simulink model "BDA_DynamicModel"  (R2021b)
settings: Solver=ode23t  StartTime=0.0  StopTime=10  FixedStep=0.000001  MaxStep=1e-5  MinStep=1e-7  RelTol=1e-3
undefined symbols (not defined in the file or in its folder): X, Y, Z
libraries: sm_lib x47, nesl_utility x7
(part 3 of 3)

== matlab function BDA_DynamicModel/H ==
  data: q2 input; H output; q3 input; q4 input; q5 input; q6 input
function H = H(q2,q3,q4,q5,q6)
%#codegen

%    This function was generated by the Symbolic Math Toolbox version 9.0.
%    01-Nov-2021 22:23:37

t2 = conj(q2);
t3 = conj(q3);
t4 = conj(q4);
t5 = conj(q5);
t6 = conj(q6);
t7 = cos(q2);
t8 = cos(q4);
t9 = cos(q5);
t10 = cos(q6);
t11 = sin(q2);
t12 = sin(q4);
t13 = sin(q5);
t14 = sin(q6);
t33 = 9.007199254740992e+15;
t15 = cos(t2);
t16 = cos(t4);
t17 = cos(t5);
t18 = cos(t6);
t19 = sin(t2);
t20 = sin(t4);
t21 = sin(t5);
t22 = sin(t6);
t25 = t7.*1.051339e-1;
t26 = t11.*1.051339e-1;
t27 = t9.*5.110348748545983e-1;
t29 = t13.*5.110348748545983e-1;
t32 = t11.*3.235525e-2;
t37 = t7.*3.235525e-2;
t40 = t9.*t12.*8.595599785252598e-1;
t41 = t12.*t13.*8.595599785252598e-1;
t55 = t9.*5.7e-7;
t56 = t10.*9.3e-7;
t57 = t14.*1.02e-6;
t63 = t13.*2.4e-7;
t65 = t9.*t14.*9.3e-7;
t66 = t14.*9.0e-8;
t67 = t13.*5.110348748545983e-9;
t68 = t10.*t13.*4.36041e-5;
t69 = t13.*t14.*4.36041e-5;
t70 = t9.*4.0e-8;
t71 = t13.*4.0e-8;
t72 = t10.*9.0e-8;
t73 = t9.*t10.*1.02e-6;
t75 = t8.*8.595599785252598e-9;
t79 = t9.*t12.*8.595599785252598e-9;
t82 = (q3.*t33)./9.007199254740992e+15;
t83 = (t3.*t33)./9.007199254740992e+15;
t88 = q3.*t33.*1.110223024625157e-16i;
t89 = t3.*t33.*1.110223024625157e-16i;
t114 = t10.*1.33637554986e-4;
t115 = t13.*1.33637554986e-4;
t117 = t13.*7.26350557185e-5;
t118 = t14.*7.26350557185e-5;
t119 = t13.*6.1855407534e-5;
t123 = t9.*1.35652563578e-4;
t127 = t9.*2.912898786671211e-7;
t131 = t8.*5.329271866856611e-7;
t134 = t9.*t10.*7.26350557185e-5;
t135 = t8.*2.784974330421842e-6;
t136 = t13.*5.212555723516903e-7;
t138 = t8.*6.730354631852784e-6;
t139 = t8.*3.748033925961328e-5;
t140 = t9.*t14.*1.33637554986e-4;
t150 = t13.*1.226483699651036e-7;
t151 = t9.*2.044139499418393e-8;
t152 = t13.*2.044139499418393e-8;
t156 = t12.*t13.*4.899491877593981e-7;
t158 = t8.*t10.*7.993907800284916e-7;
t161 = t9.*t12.*8.76751178095765e-7;
t162 = t8.*t14.*8.76751178095765e-7;
t163 = t9.*t12.*2.062943948460623e-7;
t169 = t9.*t12.*3.438239914101039e-8;
t171 = t12.*t13.*3.438239914101039e-8;
t172 = t8.*t10.*7.736039806727338e-8;
t173 = t8.*t14.*7.736039806727338e-8;
t211 = t13.*3.161027044821787e-5;
t213 = t13.*3.711904660916042e-5;
t214 = t9.*6.932319085178867e-5;
t215 = t8.*9.395517395143932e-4;
t216 = t12.*9.395517395143932e-4;
t217 = t9.*3.601891949238275e-7;
t218 = t13.*3.601891949238275e-7;
t219 = t8.*5.316843277159623e-5;
t220 = t12.*1.451749445763287e-4;
t222 = t8.*1.166015146360021e-4;
t224 = t13.*6.829345118814501e-5;
t227 = t12.*5.427853659906482e-4;
t228 = t8.*t10.*1.148694938939344e-4;
t229 = t9.*t12.*6.243418693357491e-5;
t230 = t8.*t14.*6.243418693357491e-5;
t231 = t9.*t12.*1.148694938939344e-4;
t232 = t9.*t12.*5.316843277159623e-5;
t233 = t12.*t13.*1.166015146360021e-4;
t234 = t8.*t9.*5.427853659906482e-4;
t235 = t8.*t13.*5.427853659906482e-4;
t236 = t9.*t12.*6.058377458913066e-7;
t237 = t12.*t13.*6.058377458913066e-7;
t238 = t8.*1.607033050476913e-7;
t239 = t8.*t9.*3.626595104792852e-4;
t240 = t10.*t12.*3.626595104792852e-4;
t241 = t12.*t14.*3.626595104792852e-4;
t243 = t8.*t10.*t13.*3.626595104792852e-4;
t244 = t8.*t13.*t14.*3.626595104792852e-4;
t23 = t18.*t21.*(3.0./5.0e+2);
t24 = t21.*t22.*(3.0./5.0e+2);
t28 = -t26;
t30 = t15.*1.051339e-1;
t31 = t19.*1.051339e-1;
t34 = t17.*5.110348748545983e-1;
t36 = t21.*5.110348748545983e-1;
t38 = t15.*3.235525e-2;
t39 = t19.*3.235525e-2;
t42 = t21.*9.99471e-3;
t43 = t22.*9.99471e-3;
t44 = t18.*1.838876e-2;
t45 = t21.*1.838876e-2;
t46 = t17.*1.247162e-2;
t47 = t21.*5.68686e-3;
t48 = -t41;
t50 = t16.*5.157359871151559e-3;
t51 = t16.*t18.*8.595599785252598e-1;
t52 = t17.*t20.*8.595599785252598e-1;
t53 = t16.*t22.*8.595599785252598e-1;
t54 = t20.*t21.*8.595599785252598e-1;
t58 = t17.*t18.*9.99471e-3;
t59 = t17.*t22.*1.838876e-2;
t62 = -t57;
t74 = -t66;
t76 = -t75;
t77 = t9.*t72;
t78 = t9.*t66;
t84 = cos(t82);
t85 = sin(t82);
t86 = cos(t83);
t87 = sin(t83);
t90 = exp(t88);
t91 = -t88;
t92 = -t89;
t96 = exp(t89);
t105 = t17.*6.373432765934105e-3;
t106 = t21.*5.107645374058002e-3;
t107 = t21.*2.906183788415621e-3;
t108 = t16.*3.251444605336828e-2;
t109 = t20.*3.251444605336828e-2;
t110 = t16.*1.07201054193752e-2;
t111 = t21.*9.397297665331243e-3;
t112 = t21.*3.311505989057797e-5;
t116 = t16.*4.888197259476159e-3;
t120 = t20.*5.023973353684009e-3;
t121 = t20.*4.990257941055339e-2;
t122 = t17.*3.311505989057797e-5;
t125 = t25+t32;
t126 = -t119;
t130 = t16.*t18.*1.580624215070616e-2;
t132 = t20.*t21.*1.07201054193752e-2;
t133 = t17.*t20.*1.580624215070616e-2;
t141 = t17.*t20.*8.5910527129662e-3;
t142 = t16.*t22.*8.5910527129662e-3;
t143 = t16.*t21.*4.990257941055339e-2;
t145 = -t131;
t148 = t16.*5.561353061058431e-6;
t149 = t17.*t20.*4.888197259476159e-3;
t153 = t16.*t17.*4.990257941055339e-2;
t154 = -t140;
t157 = t29+t40;
t159 = t17.*t20.*5.569948660843684e-5;
t160 = t20.*t21.*5.569948660843684e-5;
t164 = -t156;
t167 = -t162;
t174 = t16.*t18.*t21.*(-4.990257941055339e-2);
t175 = -t171;
t177 = -t173;
t184 = t55+t71;
t187 = t63+t70;
t223 = -t214;
t225 = -t217;
t226 = -t218;
t242 = -t236;
t245 = -t243;
t246 = t69+t117;
t247 = t68+t115;
t282 = t135+1.589318460797801e-6;
t283 = t138+1.655752994528898e-6;
t300 = t136+t161;
t338 = t114+t118+4.36041e-5;
t380 = t215-8.631097478604537e-5;
t381 = t216+9.554306323645785e-8;
t384 = t220+t238;
t35 = -t31;
t49 = -t47;
t60 = -t53;
t61 = -t54;
t64 = -t59;
t80 = t24+t42;
t81 = t23+t45;
t93 = 1.0./t90;
t94 = t8.*t84;
t95 = t12.*t84;
t97 = exp(t92);
t98 = t16.*t86;
t99 = t20.*t86;
t100 = t90-1.0;
t113 = -t105;
t124 = -t112;
t129 = -t122;
t137 = t28+t37;
t144 = t18.*t121;
t146 = t22.*t121;
t147 = t30+t39;
t165 = t27+t48;
t166 = -t159;
t168 = t18.*t143;
t170 = t22.*t143;
t176 = t36+t52;
t180 = t43+t44+3.0./5.0e+2;
t188 = t56+t74;
t189 = t62+t72;
t190 = t65+t77;
t191 = t73+t78;
t192 = t84.*1.273194e-2;
t193 = t86.*1.273194e-2;
t194 = t86.*1.025512e-2;
t196 = t86.*9.224950000000001e-3;
t248 = t10.*t157.*4.36041e-5;
t249 = t14.*t157.*4.36041e-5;
t258 = t84.*3.42298471896e-5;
t260 = t84.*3.07913148585e-5;
t261 = t90.*3.694216783411725e-1;
t262 = t90.*1.305783216588275e-1;
t264 = t84.*3.679077402936e-4;
t265 = t96.*1.305783216588275e-1;
t266 = t96.*3.694216783411725e-1;
t280 = t108-2.986906857247653e-3;
t281 = t109+3.306395640309251e-6;
t284 = t123+t126;
t285 = t120+t148;
t286 = t8.*t33.*t85.*5.673626844500105e-17;
t287 = t12.*t33.*t85.*5.673626844500105e-17;
t288 = t9.*t33.*t85.*9.543032792050485e-17;
t289 = t13.*t33.*t85.*9.543032792050485e-17;
t294 = t134+t154;
t296 = t16.*t33.*t87.*5.673626844500105e-17;
t297 = t20.*t33.*t87.*5.673626844500105e-17;
t298 = t17.*t33.*t87.*9.543032792050485e-17;
t299 = t21.*t33.*t87.*9.543032792050485e-17;
t303 = t16.*t33.*t87.*3.404176106700063e-19;
t304 = t8.*t33.*t85.*5.673626844500105e-25;
t305 = t13.*t33.*t85.*9.543032792050485e-25;
t306 = t84.*t86.*2.2e-7;
t307 = t90.*3.215186923359161e-3;
t309 = t90.*1.345257168956303e-2;
t310 = t96.*3.215186923359161e-3;
t311 = t96.*1.345257168956303e-2;
t319 = t67+t79+t145;
t322 = t33.*t85.*4.87211480085e-18;
t323 = t33.*t87.*4.87211480085e-18;
t324 = t33.*t87.*6.374153504905841e-18;
t325 = t12.*t33.*t85.*5.582848814988104e-22;
t327 = t33.*t87.*5.577730892363251e-19;
t328 = t8.*t33.*t85.*2.479366200131245e-18;
t329 = t21.*t33.*t87.*9.537984527703491e-19;
t330 = t8.*t33.*t85.*7.351481000981246e-18;
t331 = t8.*t33.*t85.*4.442449819243582e-22;
t332 = t12.*t33.*t85.*9.810473427588925e-18;
t333 = t12.*t33.*t85.*4.938358626738924e-18;
t334 = t8.*t33.*t85.*3.517648643590065e-23;
t335 = t33.*t85.*3.091942624624357e-22;
t336 = t16.*t33.*t87.*2.479366200131245e-18;
t337 = t8.*t33.*t85.*1.838255097618034e-22;
t339 = t16.*t33.*t87.*3.226512155691387e-19;
t342 = t21.*t33.*t87.*5.426989146380022e-19;
t343 = t33.*t85.*2.967883198327701e-22;
t344 = t20.*t33.*t87.*3.31613276532711e-19;
t345 = t17.*t33.*t87.*1.190170786299927e-18;
t346 = t21.*t33.*t87.*1.754845396851463e-18;
t348 = t16.*t33.*t87.*7.075931802640439e-19;
t349 = t20.*t33.*t87.*4.938358626738924e-18;
t350 = t33.*t87.*6.174342216456664e-22;
t352 = t16.*t33.*t87.*8.66274921222547e-18;
t354 = t16.*t33.*t87.*3.790634411375469e-18;
t355 = t20.*t33.*t87.*8.66274921222547e-18;
t357 = t20.*t33.*t87.*3.790634411375469e-18;
t358 = t8.*t33.*t85.*2.47393392290267e-21;
t359 = t16.*t33.*t87.*7.351481000981246e-18;
t360 = t20.*t33.*t87.*9.810473427588925e-18;
t362 = t9.*t33.*t85.*5.439528691468777e-23;
t363 = t17.*t33.*t87.*6.183885249248715e-21;
t364 = t21.*t33.*t87.*6.183885249248715e-21;
t365 = t13.*t33.*t85.*9.733893447891495e-23;
t369 = t13.*t33.*t85.*2.290327870092116e-23;
t370 = t16.*t33.*t87.*3.670836568391568e-22;
t372 = t9.*t33.*t85.*3.817213116820194e-24;
t373 = t13.*t33.*t85.*3.817213116820194e-24;
t374 = t90.*1.073174736839591e-5;
t375 = t90.*4.490239736257417e-5;
t378 = t90.*3.887314306731568e-4;
t382 = t33.*t85.*2.127584079327986e-20;
t386 = t33.*t85.*1.611765660673211e-20;
t387 = t13.*t33.*t85.*6.931587185740596e-21;
t388 = t8.*t33.*t85.*7.696420262413979e-21;
t389 = t8.*t33.*t85.*3.509445006623964e-21;
t390 = t9.*t33.*t85.*1.294536862550567e-20;
t391 = t12.*t33.*t85.*5.371403294717661e-20;
t392 = t8.*t33.*t85.*9.394124637620594e-23;
t395 = t13.*t33.*t85.*1.275307569480848e-20;
t397 = t12.*t33.*t85.*9.582443148530891e-21;
t398 = t13.*t33.*t85.*5.902881824626087e-21;
t401 = t9.*t33.*t85.*6.726150146755334e-23;
t402 = t13.*t33.*t85.*6.726150146755334e-23;
t404 = t33.*t85.*1.78416509397307e-23;
t405 = t8.*t33.*t85.*2.503226128461205e-19;
t406 = t12.*t33.*t85.*2.503226128461205e-19;
t407 = t8.*t33.*t85.*1.095358398302466e-19;
t409 = t12.*t33.*t85.*1.06707538424542e-19;
t410 = t12.*t33.*t85.*1.095358398302466e-19;
t415 = t8.*t33.*t85.*1.060741086483328e-23;
t419 = t33.*t85.*t125.*5.673626844500105e-17;
t424 = t85.*t87.*7.913131956031502e-8;
t434 = t13.*t33.*t85.*4.011313864537747e-22;
t435 = t9.*t33.*t85.*3.825067422357704e-25;
t436 = t8.*t33.*t85.*1.511210377393976e-22;
t438 = t33.*t85.*t125.*1.893760189037778e-19;
t439 = t21.*t33.*t87.*4.011313864537747e-22;
t440 = t17.*t33.*t87.*3.825067422357704e-25;
t441 = t16.*t33.*t87.*1.511210377393976e-22;
t471 = t33.*t85.*3.909932369564116e-22;
t472 = t13.*t33.*t85.*1.793163166137816e-24;
t473 = t33.*t87.*3.909932369564116e-22;
t474 = t21.*t33.*t87.*1.793163166137816e-24;
t481 = t33.*t85.*9.467866758889686e-23;
t482 = t33.*t87.*5.699051429514929e-23;
t498 = t33.*t87.*t282.*9.543032792050485e-17;
t505 = t127+t152+t164+t169;
t523 = t76+t150+t151+t163+t175;
t557 = t219+t225+t234+t237;
t558 = t222+t226+t235+t242;
t583 = t211+t223+t227+t232+t233;
t101 = t100.^2;
t102 = t97-1.0;
t104 = t99.*(3.0./5.0e+2);
t128 = t95./1.0e+8;
t155 = t35+t38;
t178 = t34+t61;
t179 = t46+t49;
t183 = t58+t64;
t185 = t18.*t176.*(3.0./5.0e+2);
t186 = t22.*t176.*(3.0./5.0e+2);
t195 = t95.*2.228474e-2;
t197 = t94.*6.562549e-2;
t198 = t94.*9.840000000000001e-6;
t199 = t98.*4.539638e-2;
t200 = t99.*4.539638e-2;
t201 = t99.*1.247162e-2;
t202 = t99.*2.228474e-2;
t203 = t98.*5.84482e-3;
t204 = t98.*6.562549e-2;
t205 = t99.*5.68686e-3;
t207 = t95.*3.24e-6;
t208 = t95.*7.83e-6;
t209 = t95.*4.36041e-5;
t210 = t95.*6.2e-7;
t212 = t99.*6.47e-6;
t251 = t10.*t165.*1.02e-6;
t252 = t14.*t165.*9.3e-7;
t255 = t72.*t165;
t256 = t66.*t165;
t263 = t93.*3.694216783411725e-1;
t267 = t93.*1.305783216588275e-1;
t268 = t97.*1.305783216588275e-1;
t269 = t97.*3.694216783411725e-1;
t270 = t94.*1.3117937708872e-3;
t271 = t95.*1.3117937708872e-3;
t272 = t95.*1.35652563578e-4;
t273 = t94.*1.688944904408e-4;
t274 = t95.*6.1855407534e-5;
t275 = t94.*7.13801892181e-4;
t276 = t95.*1.655752994528898e-6;
t277 = t95.*1.869599668e-7;
t290 = t14.*t165.*1.33637554986e-4;
t291 = t10.*t165.*7.26350557185e-5;
t292 = -t287;
t293 = -t288;
t301 = -t297;
t302 = -t298;
t308 = t93.*3.215186923359161e-3;
t312 = t93.*1.345257168956303e-2;
t313 = t97.*3.215186923359161e-3;
t314 = t97.*1.345257168956303e-2;
t315 = t95.*4.427198467956924e-6;
t316 = t95.*2.663570267859459e-6;
t317 = t99.*4.427198467956924e-6;
t318 = t99.*2.663570267859459e-6;
t320 = t94.*8.487305697640184e-9;
t321 = t98.*8.487305697640184e-9;
t326 = -t325;
t340 = -t332;
t341 = -t333;
t347 = -t335;
t351 = -t343;
t353 = -t344;
t356 = -t345;
t361 = -t349;
t366 = -t355;
t367 = -t357;
t368 = -t360;
t371 = -t370;
t376 = t93.*1.073174736839591e-5;
t377 = t93.*4.490239736257417e-5;
t379 = t93.*3.887314306731568e-4;
t383 = t95+t286;
t396 = t99+t296;
t399 = -t390;
t400 = -t391;
t403 = -t392;
t411 = -t397;
t412 = -t406;
t413 = -t409;
t414 = -t410;
t416 = -t415;
t420 = t33.*t85.*t137.*9.543032792050485e-17;
t425 = t33.*t87.*t147.*5.673626844500105e-17;
t442 = t33.*t85.*t137.*3.185302114428987e-19;
t483 = -t482;
t499 = t116+t129+t153+t160;
t500 = t110+t124+t143+t166;
t526 = t107+t113+t121+t132+t149;
t585 = t213+t229+t241+t245+t249;
t586 = t224+t231+t240+t244+t248;
t103 = t102.^2;
t181 = t18.*t178;
t182 = t22.*t178;
t206 = -t204;
t221 = -t212;
t278 = -t276;
t279 = -t277;
t295 = -t291;
t385 = t94+t292;
t408 = t98+t301;
t417 = t18.*t396;
t418 = t22.*t396;
t423 = -t420;
t426 = t33.*t87.*t155.*9.543032792050485e-17;
t428 = t93.*t101.*7.997968101822611e-3;
t430 = t93.*t101.*5.407940120688672e-3;
t433 = (t13.*t396)./1.0e+8;
t437 = t13.*t383.*4.334075e-2;
t443 = t56.*t383;
t444 = t57.*t383;
t445 = -t442;
t446 = t43.*t396;
t447 = t44.*t396;
t450 = t14.*t383.*(-1.02e-6);
t451 = t17.*t396.*4.334075e-2;
t452 = t21.*t396.*4.334075e-2;
t455 = t72.*t383;
t456 = t66.*t383;
t460 = t14.*t383.*(-9.0e-8);
t461 = t93.*t101.*2.669585786930656e-5;
t465 = t93.*t101.*1.805078477303827e-5;
t470 = t93.*t101.*1.56270217221073e-4;
t475 = t93.*t101.*t125.*2.196325630278387e-1;
t476 = t93.*t101.*t137.*2.196325630278387e-1;
t484 = t198+t326;
t485 = t9.*t383.*4.71413003675e-4;
t486 = t13.*t383.*4.71413003675e-4;
t487 = t114.*t383;
t488 = t9.*t383.*3.149723995125e-4;
t489 = t118.*t383;
t501 = t93.*t101.*t125.*7.330961578512107e-4;
t502 = t93.*t101.*t137.*7.330961578512107e-4;
t503 = t93.*t101.*t125.*6.346599179580158e-3;
t506 = t13.*t383.*5.879283844893203e-6;
t507 = t9.*t383.*2.68085975407921e-6;
t512 = t21.*t396.*5.879283844893203e-6;
t513 = t17.*t396.*2.68085975407921e-6;
t515 = t261+t263+2.61156643317655e-1;
t516 = t262+t267+7.38843356682345e-1;
t519 = t265+t268+7.38843356682345e-1;
t520 = t266+t269+2.61156643317655e-1;
t524 = t283.*t396;
t536 = t319.*t396;
t537 = t111+t133+t144+t170+t185;
t538 = t106+t141+t146+t174+t186;
t539 = t158+t177+t252+t255;
t540 = t167+t172+t251+t256;
t576 = t208+t331+t347;
t577 = t207+t337+t351;
t250 = t182.*1.838876e-2;
t253 = t181.*9.99471e-3;
t257 = t51+t182;
t259 = t60+t181;
t393 = t9.*t385;
t394 = t13.*t385;
t421 = t17.*t408;
t422 = t21.*t408;
t427 = -t426;
t431 = t96.*t103.*7.997968101822611e-3;
t432 = t96.*t103.*5.407940120688672e-3;
t463 = t70.*t385;
t464 = t71.*t385;
H = ft_1({t10,t103,t104,t11,t114,t118,t119,t12,t123,t125,t128,t13,t130,t137,t139,t14,t142,t147,t15,t153,t155,t157,t16,t17,t176,t178,t179,t18,t180,t181,t183,t184,t187,t188,t189,t19,t190,t191,t192,t193,t194,t195,t196,t197,t199,t20,t200,t201,t202,t203,t204,t205,t206,t209,t21,t210,t218,t22,t221,t222,t228,t230,t235,t236,t239,t246,t247,t250,t253,t257,t258,t260,t264,t270,t271,t272,t273,t274,t275,t278,t279,t280,t281,t283,t285,t288,t289,t290,t293,t294,t295,t298,t299,t300,t302,t303,t304,t305,t306,t307,t308,t309,t31,t310,t311,t312,t313,t314,t315,t316,t317,t318,t319,t320,t321,t322,t323,t324,t327,t328,t329,t33,t330,t334,t336,t338,t339,t340,t341,t342,t346,t348,t349,t350,t352,t353,t354,t356,t358,t359,t361,t362,t363,t364,t365,t366,t367,t368,t369,t371,t372,t373,t374,t375,t376,t377,t378,t379,t38,t380,t381,t382,t383,t384,t386,t387,t388,t389,t393,t394,t395,t396,t398,t399,t400,t401,t402,t403,t404,t405,t407,t408,t411,t412,t413,t414,t416,t417,t418,t419,t421,t422,t423,t424,t425,t427,t428,t430,t431,t432,t433,t434,t435,t436,t437,t438,t439,t440,t441,t443,t445,t446,t447,t450,t451,t452,t455,t460,t461,t463,t465,t470,t471,t472,t473,t474,t475,t476,t481,t483,t484,t485,t486,t487,t488,t489,t498,t499,t50,t500,t501,t502,t503,t505,t506,t507,t512,t513,t515,t516,t519,t520,t523,t524,t526,t53,t536,t537,t538,t539,t540,t557,t576,t577,t583,t585,t586,t66,t7,t72,t8,t80,t81,t85,t87,t9,t96});
end
function H = ft_1(ct)
t10 = ct{1};
t103 = ct{2};
t104 = ct{3};
t11 = ct{4};
t114 = ct{5};
t118 = ct{6};
t119 = ct{7};
t12 = ct{8};
t123 = ct{9};
t125 = ct{10};
t128 = ct{11};
t13 = ct{12};
t130 = ct{13};
t137 = ct{14};
t139 = ct{15};
t14 = ct{16};
t142 = ct{17};
t147 = ct{18};
t15 = ct{19};
t153 = ct{20};
t155 = ct{21};
t157 = ct{22};
t16 = ct{23};
t17 = ct{24};
t176 = ct{25};
t178 = ct{26};
t179 = ct{27};
t18 = ct{28};
t180 = ct{29};
t181 = ct{30};
t183 = ct{31};
t184 = ct{32};
t187 = ct{33};
t188 = ct{34};
t189 = ct{35};
t19 = ct{36};
t190 = ct{37};
t191 = ct{38};
t192 = ct{39};
t193 = ct{40};
t194 = ct{41};
t195 = ct{42};
t196 = ct{43};
t197 = ct{44};
t199 = ct{45};
t20 = ct{46};
t200 = ct{47};
t201 = ct{48};
t202 = ct{49};
t203 = ct{50};
t204 = ct{51};
t205 = ct{52};
t206 = ct{53};
t209 = ct{54};
t21 = ct{55};
t210 = ct{56};
t218 = ct{57};
t22 = ct{58};
t221 = ct{59};
t222 = ct{60};
t228 = ct{61};
t230 = ct{62};
t235 = ct{63};
t236 = ct{64};
t239 = ct{65};
t246 = ct{66};
t247 = ct{67};
t250 = ct{68};
t253 = ct{69};
t257 = ct{70};
t258 = ct{71};
t260 = ct{72};
t264 = ct{73};
t270 = ct{74};
t271 = ct{75};
t272 = ct{76};
t273 = ct{77};
t274 = ct{78};
t275 = ct{79};
t278 = ct{80};
t279 = ct{81};
t280 = ct{82};
t281 = ct{83};
t283 = ct{84};
t285 = ct{85};
t288 = ct{86};
t289 = ct{87};
t290 = ct{88};
t293 = ct{89};
t294 = ct{90};
t295 = ct{91};
t298 = ct{92};
t299 = ct{93};
t300 = ct{94};
t302 = ct{95};
t303 = ct{96};
t304 = ct{97};
t305 = ct{98};
t306 = ct{99};
t307 = ct{100};
t308 = ct{101};
t309 = ct{102};
t31 = ct{103};
t310 = ct{104};
t311 = ct{105};
t312 = ct{106};
t313 = ct{107};
t314 = ct{108};
t315 = ct{109};
t316 = ct{110};
t317 = ct{111};
t318 = ct{112};
t319 = ct{113};
t320 = ct{114};
t321 = ct{115};
t322 = ct{116};
t323 = ct{117};
t324 = ct{118};
t327 = ct{119};
t328 = ct{120};
t329 = ct{121};
t33 = ct{122};
t330 = ct{123};
t334 = ct{124};
t336 = ct{125};
t338 = ct{126};
t339 = ct{127};
t340 = ct{128};
t341 = ct{129};
t342 = ct{130};
t346 = ct{131};
t348 = ct{132};
t349 = ct{133};
t350 = ct{134};
t352 = ct{135};
t353 = ct{136};
t354 = ct{137};
t356 = ct{138};
t358 = ct{139};
t359 = ct{140};
t361 = ct{141};
t362 = ct{142};
t363 = ct{143};
t364 = ct{144};
t365 = ct{145};
t366 = ct{146};
t367 = ct{147};
t368 = ct{148};
t369 = ct{149};
t371 = ct{150};
t372 = ct{151};
t373 = ct{152};
t374 = ct{153};
t375 = ct{154};
t376 = ct{155};
t377 = ct{156};
t378 = ct{157};
t379 = ct{158};
t38 = ct{159};
t380 = ct{160};
t381 = ct{161};
t382 = ct{162};
t383 = ct{163};
t384 = ct{164};
t386 = ct{165};
t387 = ct{166};
t388 = ct{167};
t389 = ct{168};
t393 = ct{169};
t394 = ct{170};
t395 = ct{171};
t396 = ct{172};
t398 = ct{173};
t399 = ct{174};
t400 = ct{175};
t401 = ct{176};
t402 = ct{177};
t403 = ct{178};
t404 = ct{179};
t405 = ct{180};
t407 = ct{181};
t408 = ct{182};
t411 = ct{183};
t412 = ct{184};
t413 = ct{185};
t414 = ct{186};
t416 = ct{187};
t417 = ct{188};
t418 = ct{189};
t419 = ct{190};
t421 = ct{191};
t422 = ct{192};
t423 = ct{193};
t424 = ct{194};
t425 = ct{195};
t427 = ct{196};
t428 = ct{197};
t430 = ct{198};
t431 = ct{199};
t432 = ct{200};
t433 = ct{201};
t434 = ct{202};
t435 = ct{203};
t436 = ct{204};
t437 = ct{205};
t438 = ct{206};
t439 = ct{207};
t440 = ct{208};
t441 = ct{209};
t443 = ct{210};
t445 = ct{211};
t446 = ct{212};
t447 = ct{213};
t450 = ct{214};
t451 = ct{215};
t452 = ct{216};
t455 = ct{217};
t460 = ct{218};
t461 = ct{219};
t463 = ct{220};
t465 = ct{221};
t470 = ct{222};
t471 = ct{223};
t472 = ct{224};
t473 = ct{225};
t474 = ct{226};
t475 = ct{227};
t476 = ct{228};
t481 = ct{229};
t483 = ct{230};
t484 = ct{231};
t485 = ct{232};
t486 = ct{233};
t487 = ct{234};
t488 = ct{235};
t489 = ct{236};
t498 = ct{237};
t499 = ct{238};
t50 = ct{239};
t500 = ct{240};
t501 = ct{241};
t502 = ct{242};
t503 = ct{243};
t505 = ct{244};
t506 = ct{245};
t507 = ct{246};
t512 = ct{247};
t513 = ct{248};
t515 = ct{249};
t516 = ct{250};
t519 = ct{251};
t520 = ct{252};
t523 = ct{253};
t524 = ct{254};
t526 = ct{255};
t53 = ct{256};
t536 = ct{257};
t537 = ct{258};
t538 = ct{259};
t539 = ct{260};
t540 = ct{261};
t557 = ct{262};
t576 = ct{263};
t577 = ct{264};
t583 = ct{265};
t585 = ct{266};
t586 = ct{267};
t66 = ct{268};
t7 = ct{269};
t72 = ct{270};
t8 = ct{271};
t80 = ct{272};
t81 = ct{273};
t85 = ct{274};
t87 = ct{275};
t9 = ct{276};
t96 = ct{277};
t477 = -t476;
t478 = t96.*t103.*t147.*2.196325630278387e-1;
t479 = t96.*t103.*t155.*2.196325630278387e-1;
t497 = t12.*t408.*8.458070188688557e-6;
t504 = -t502;
t509 = t20.*t484.*8.595599785252598e-1;
t525 = -t524;
t541 = t125.*t516;
t542 = t137.*t515;
t544 = t147.*t519;
t545 = t155.*t520;
t578 = t408.*t484;
t580 = t16.*t576.*8.595599785252598e-1;
t589 = t33.*t87.*t577.*9.543032792050485e-17;
t591 = t322+t419+t423;
t600 = t307+t308+t428+1.819229615328168e-2;
t617 = t396.*t576;
t624 = t139+t228+t230+t239+t290+t295;
t627 = t382+t438+t445;
t629 = t192+t309+t312+t430+9.510076620873934e-3;
t646 = t260+t374+t376+t461+6.072279186930818e-5;
t647 = t258+t375+t377+t465+3.174301904745164e-5;
t713 = t264+t273+t279+t378+t379+t411+t416+t470+2.748073584704864e-4;
t254 = -t253;
t429 = t393./1.0e+8;
t448 = t394.*5.7e-7;
t449 = t393.*1.02e-6;
t453 = t421.*9.99471e-3;
t454 = t421.*1.838876e-2;
t458 = t393.*2.4e-7;
t459 = t422.*1.247162e-2;
t462 = t421.*5.68686e-3;
t466 = t421.*6.48e-5;
t467 = t422.*6.48e-5;
t468 = t394.*(-4.0e-8);
t480 = -t479;
t490 = t394.*1.35652563578e-4;
t491 = t393.*1.33637554986e-4;
t492 = t393.*7.26350557185e-5;
t493 = t393.*6.1855407534e-5;
t494 = t393.*7.0482312e-7;
t495 = t394.*7.0482312e-7;
t508 = t393.*4.203395243364607e-6;
t510 = t394.*4.0082304082032e-9;
t514 = t421.*4.203395243364607e-6;
t517 = t422.*4.0082304082032e-9;
t521 = t393.*1.87902861198544e-8;
t522 = t421.*1.87902861198544e-8;
t527 = t289+t393;
t528 = t293+t394;
t529 = t299+t421;
t530 = t302+t422;
t531 = -t18.*(t298-t422);
t532 = -t22.*(t298-t422);
t533 = t18.*(t298-t422);
t543 = -t542;
t546 = -t545;
t549 = t10.*(t288-t394).*(-1.02e-6);
t550 = t14.*(t288-t394).*(-9.3e-7);
t551 = -t72.*(t288-t394);
t552 = -t66.*(t288-t394);
t554 = t22.*(t298-t422).*(-1.838876e-2);
t559 = t541.*3.33783e-3;
t560 = t542.*3.33783e-3;
t561 = t542.*2.889644e-2;
t564 = t14.*(t288-t394).*(-1.33637554986e-4);
t566 = t10.*(t288-t394).*(-7.26350557185e-5);
t567 = t10.*(t288-t394).*7.26350557185e-5;
t573 = -t184.*(t298-t422);
t575 = t184.*(t298-t422);
t581 = -t580;
t590 = -t589;
t592 = t8.*t591;
t593 = t12.*t591;
t595 = t323+t425+t427;
t596 = t324+t425+t427;
t601 = t8.*t600;
t602 = t12.*t600;
t603 = t310+t313+t431+1.819229615328168e-2;
t612 = -t505.*(t298-t422);
t613 = t505.*(t298-t422);
t630 = t9.*t629;
t632 = t194+t311+t314+t432+9.510076620873934e-3;
t633 = t193+t311+t314+t432+9.510076620873934e-3;
t637 = t13.*t629.*7.26735e-3;
t639 = t13.*t629.*1.08769e-2;
t675 = t477+t541+t600;
t685 = -t18.*(-t443+t14.*t383.*9.0e-8+t14.*(t288-t394).*9.3e-7+t72.*(t288-t394));
t686 = -t22.*(-t455+t14.*t383.*1.02e-6+t10.*(t288-t394).*1.02e-6+t66.*(t288-t394));
t687 = t22.*(-t455+t14.*t383.*1.02e-6+t10.*(t288-t394).*1.02e-6+t66.*(t288-t394));
t688 = -t17.*t18.*(-t455+t14.*t383.*1.02e-6+t10.*(t288-t394).*1.02e-6+t66.*(t288-t394));
t689 = -t17.*t22.*(-t443+t14.*t383.*9.0e-8+t14.*(t288-t394).*9.3e-7+t72.*(t288-t394));
t690 = t17.*t18.*(-t455+t14.*t383.*1.02e-6+t10.*(t288-t394).*1.02e-6+t66.*(t288-t394));
t691 = t17.*t22.*(-t443+t14.*t383.*9.0e-8+t14.*(t288-t394).*9.3e-7+t72.*(t288-t394));
t708 = -t257.*(-t443+t14.*t383.*9.0e-8+t14.*(t288-t394).*9.3e-7+t72.*(t288-t394));
t709 = (t53-t181).*(-t455+t14.*t383.*1.02e-6+t10.*(t288-t394).*1.02e-6+t66.*(t288-t394));
t710 = t257.*(-t443+t14.*t383.*9.0e-8+t14.*(t288-t394).*9.3e-7+t72.*(t288-t394));
t457 = -t448;
t469 = -t467;
t496 = -t495;
t511 = -t510;
t518 = -t517;
t534 = t18.*t529.*(3.0./5.0e+2);
t535 = t22.*t529.*(3.0./5.0e+2);
t547 = t10.*t527.*4.36041e-5;
t548 = t14.*t527.*4.36041e-5;
t553 = t533.*(-9.99471e-3);
t555 = t533.*9.99471e-3;
t556 = t13.*t529.*1.02e-6;
t562 = -t560;
t563 = -t561;
t565 = t14.*t527.*4.35810334311e-7;
t568 = t10.*t527.*8.01825329916e-7;
t569 = t365+t449;
t571 = t22.*t529.*4.35810334311e-7;
t572 = t18.*t529.*8.01825329916e-7;
t574 = t187.*t529;
t579 = t50+t130+t142+t153+t250+t254;
t584 = t300.*t529;
t587 = t417+t532;
t588 = t418+t533;
t594 = -t593;
t597 = t16.*t595;
t598 = t20.*t595;
t604 = t16.*t603;
t605 = t20.*t603;
t606 = t592.*2.889644e-2;
t607 = t593.*2.889644e-2;
t609 = t593.*1.08769e-2;
t611 = t210+t305+t334+t429;
t614 = t601.*2.889644e-2;
t615 = t602.*2.889644e-2;
t616 = t601.*1.08769e-2;
t628 = t523.*t529;
t631 = t196+t603;
t634 = t17.*t633;
t635 = t21.*t633;
t638 = t630.*1.08769e-2;
t640 = -t637;
t641 = -t639;
t648 = t195+t330+t602;
t649 = t197+t340+t601;
t666 = t128+t304+t369+t372+t458+t468;
t676 = t8.*t675;
t677 = t12.*t675;
t678 = t203+t221+t353+t371+t633;
t679 = t480+t544+t603;
t683 = t443+t460+t550+t551;
t684 = t450+t455+t549+t552;
t695 = t475+t543+t629;
t698 = t478+t546+t633;
t699 = t478+t546+t632;
t711 = -t709;
t714 = t504+t559+t646;
t570 = t21.*t569;
t582 = t176.*t569;
t599 = -t598;
t608 = -t607;
t610 = -t609;
t618 = t188.*t587;
t619 = t189.*t588;
t620 = t190.*t587;
t623 = t191.*t588;
t625 = t16.*t611.*8.595599785252598e-1;
t636 = -t635;
t642 = t529.*t569;
t643 = t396.*t611;
t644 = t362+t373+t457+t463;
t650 = t13.*t648;
t651 = t202+t359+t605;
t652 = t204+t368+t604;
t658 = t9.*t648.*7.26735e-3;
t659 = t9.*t648.*1.08769e-2;
t661 = t10.*t649.*7.26735e-3;
t662 = t14.*t649.*7.26735e-3;
t663 = t539.*t587;
t665 = t540.*t588;
t667 = t200+t327+t352+t605;
t668 = t21.*t666;
t669 = t199+t350+t366+t604;
t670 = t176.*t666;
t671 = t271+t386+t405+t615;
t672 = t270+t404+t412+t614;
t680 = t16.*t679;
t681 = t20.*t679;
t692 = t676.*2.889644e-2;
t693 = t677.*2.889644e-2;
t694 = t676.*1.08769e-2;
t696 = t9.*t695;
t697 = t480+t544+t631;
t700 = t17.*t698;
t701 = t21.*t698;
t704 = t13.*t695.*1.08769e-2;
t705 = t13.*t695.*7.26735e-3;
t712 = t529.*t666;
t715 = t501+t562+t647;
t718 = -t587.*(-t443+t14.*t383.*9.0e-8+t14.*(t288-t394).*9.3e-7+t72.*(t288-t394));
t719 = -t588.*(-t455+t14.*t383.*1.02e-6+t10.*(t288-t394).*1.02e-6+t66.*(t288-t394));
t720 = t588.*(-t455+t14.*t383.*1.02e-6+t10.*(t288-t394).*1.02e-6+t66.*(t288-t394));
t728 = t478+t546+t678;
t729 = t275+t398+t399+t413+t490+t493+t616;
t730 = t195+t328+t592+t677;
t732 = t197+t341+t594+t676;
t746 = t503+t563+t713;
t621 = -t619;
t622 = -t620;
t626 = -t625;
t645 = t17.*t644;
t653 = t17.*t651;
t654 = t21.*t651;
t655 = t18.*t652;
t656 = t22.*t652;
t657 = t650.*1.08769e-2;
t660 = t178.*t644;
t664 = -t663;
t673 = -t644.*(t298-t422);
t674 = t644.*(t298-t422);
t682 = -t680;
t702 = -t701;
t703 = t696.*1.08769e-2;
t706 = -t704;
t707 = -t705;
t716 = t342+t356+t459+t462+t652;
t717 = t437+t630+t650;
t731 = t13.*t730;
t733 = t202+t336+t597+t681;
t737 = -t18.*(t204+t361+t599+t680);
t738 = -t22.*(t204+t361+t599+t680);
t739 = t18.*(t204+t361+t599+t680);
t740 = t22.*(t204+t361+t599+t680);
t741 = t9.*t730.*7.26735e-3;
t742 = t9.*t730.*1.08769e-2;
t744 = t10.*t732.*7.26735e-3;
t745 = t14.*t732.*7.26735e-3;
t747 = t200+t327+t354+t597+t681;
t748 = t199+t350+t367+t599+t680;
t749 = t271+t386+t407+t606+t693;
t750 = t270+t404+t414+t608+t692;
t754 = t274+t389+t401+t485+t496+t641+t659;
t755 = t204+t342+t356+t361+t459+t462+t599+t680;
t756 = t275+t398+t399+t400+t490+t493+t610+t694;
t760 = t209+t358+t487+t488+t489+t564+t567+t640+t658;
t721 = t452+t634+t654;
t725 = t10.*t717.*7.26735e-3;
t726 = t14.*t717.*7.26735e-3;
t734 = t17.*t733;
t735 = t21.*t733;
t736 = t206+t349+t598+t682;
t743 = t731.*1.08769e-2;
t752 = t205+t339+t363+t451+t469+t636+t653;
t753 = t272+t388+t402+t486+t494+t638+t657;
t757 = t104+t303+t446+t447+t451+t554+t555+t636+t653;
t763 = t437+t696+t731;
t774 = t274+t389+t401+t485+t496+t706+t742;
t776 = t209+t358+t487+t488+t489+t564+t567+t707+t741;
t722 = t22.*t721;
t723 = t18.*t721;
t727 = -t726;
t751 = t201+t348+t364+t466+t721;
t761 = t387+t492+t548+t662+t725;
t764 = t10.*t763.*7.26735e-3;
t765 = t14.*t763.*7.26735e-3;
t767 = t452+t700+t735;
t772 = t205+t339+t363+t451+t469+t702+t734;
t773 = t272+t388+t402+t486+t494+t703+t743;
t775 = t104+t303+t446+t447+t451+t554+t555+t702+t734;
t724 = -t722;
t758 = t329+t453+t535+t656+t723;
t762 = t395+t491+t547+t661+t727;
t766 = -t765;
t768 = t18.*t767;
t769 = t22.*t767;
t771 = t201+t348+t364+t466+t767;
t779 = t387+t492+t548+t745+t764;
t759 = t346+t454+t534+t655+t724;
t770 = -t769;
t777 = t329+t453+t535+t740+t768;
t780 = t395+t491+t547+t744+t766;
t778 = t346+t454+t534+t739+t770;
et1 = t7.*(-6.595899203175001e-4)+t11.*2.143246017993e-3;
et2 = 4.573233567645e-4;
et3 = t147+1.580661e-2;
et4 = t7.*2.143246017993e-3+t11.*6.595899203175001e-4+3.222314966007e-4;
et5 = t7.*1.908064240151374e-5+t11.*5.850606868813307e-5+t306;
et6 = t424+t578+t590+t617+t642+t643+t674+t712+t718+t720+t324.*t627+t631.*t714+t632.*t715+t667.*t749+t669.*t750+t678.*t746+t716.*t756+t751.*t773+t752.*t774+t757.*t776+t758.*t779+t759.*t780+1.896268252195649e-5;
et7 = t278+t403+t481+t509+t581+t582+t626+t660+t670+t710+t711-t280.*t749+t281.*t750+t285.*t746-t499.*t774-t500.*t773+t526.*t756+t537.*t780+t538.*t779-t579.*t776-t33.*t85.*t125.*5.091703513734173e-22;
et8 = t33.*t85.*t137.*8.564238525144865e-22;
et9 = t315+t320+t471+t570+t592.*1.688944904408e-4-t593.*1.869599668e-7+t645+t668;
et10 = t676.*1.869599668e-7+t677.*1.688944904408e-4+t690+t691+t17.*t774.*6.48e-5;
et11 = t21.*t773.*6.48e-5+t80.*t779+t81.*t780-t179.*t756+t183.*t776;
et12 = t8.*t33.*t85.*4.563917575948183e-22;
et13 = t12.*t33.*t85.*(-7.086968837016952e-25);
et14 = t316+t435+t436+t472+t506+t507+t511+t521+t685+t687+t731.*1.35652563578e-4-t13.*t695.*6.1855407534e-5;
et15 = t9.*t730.*6.1855407534e-5+t123.*t695+t180.*t776;
et16 = t15.*1.908064240151374e-5+t19.*5.850606868813307e-5+t306;
et17 = t424+t578+t590+t617+t642+t643+t674+t712+t718+t720+t382.*t596+t646.*t697+t647.*t699+t671.*t747+t672.*t748+t713.*t728+t729.*t755+t753.*t771+t754.*t772+t760.*t775+t761.*t777+t762.*t778+1.896268252195649e-5;
et18 = t306+t578+t590+t617+t642+t643+t674+t712+t718+t720+t85.*t87.*1.108156578290307e-5+t631.*t646+t632.*t647+t667.*t671+t669.*t672+t678.*t713+t716.*t729+t751.*t753;
et19 = t752.*t754+t757.*t760+t758.*t761+t759.*t762+1.896268252195649e-5;
et20 = t315+t320+t471+t570+t601.*1.869599668e-7+t602.*1.688944904408e-4+t645+t668+t690+t691+t17.*t754.*6.48e-5;
et21 = t21.*t753.*6.48e-5+t80.*t761+t81.*t762-t179.*t729+t183.*t760;
et22 = t8.*t33.*t85.*1.279265104253459e-21;
et23 = t12.*t33.*t85.*(-1.6195873051144e-24);
et24 = t316+t435+t436+t472+t506+t507+t511+t521+t650.*1.35652563578e-4+t685+t687-t13.*t629.*6.1855407534e-5;
et25 = t9.*t648.*6.1855407534e-5+t123.*t629+t180.*t760;
et26 = t483+t497+t498+t525+t536+t584+t613+t628+t664+t665+t384.*t728-t380.*t747+t381.*t748-t557.*t772+t583.*t755+t585.*t777+t586.*t778-t624.*t775+t771.*(t218-t222-t235+t236);
et27 = t33.*t87.*t147.*(-5.091703513734173e-22);
et28 = t33.*t87.*t155.*8.564238525144865e-22;
et29 = t8.*1.423219008420395e-6;
et30 = t12.*t20.*7.270218629754276e-6+t16.*t283.*8.595599785252598e-1-t16.*t319.*8.595599785252598e-1+t176.*t300+t280.*t380+t281.*t381+t285.*t384+t178.*t505+t176.*t523+t257.*t539;
et31 = t499.*t557+t526.*t583+t537.*t586+t538.*t585+t579.*t624-t540.*(t53-t181)-t500.*(t218-t222-t235+t236);
et32 = 1.027194904463421e-6;
et33 = t8.*(-2.706536467726674e-6);
et34 = t12.*6.078899754658124e-9+t21.*t300+t17.*t505+t21.*t523-t17.*t557.*6.48e-5+t80.*t585+t81.*t586-t179.*t583;
et35 = -t183.*t624+t21.*(t218-t222-t235+t236).*6.48e-5+t17.*t18.*t540+t17.*t22.*t539;
et36 = 2.093791190610393e-6;
et37 = t8.*(-2.289498402241797e-6);
et38 = t9.*2.048345525044518e-9;
et39 = t13.*9.602491515741889e-9;
et40 = t8.*t9.*(-3.086744386437578e-6);
et41 = t8.*t13.*(-6.769412826196288e-6);
et42 = t9.*t12.*1.615137793366553e-8;
et43 = t12.*t13.*(-3.445314443599436e-9)-t18.*t539+t22.*t540-t180.*t624;
et44 = t13.*2.148081562157245e-6;
et45 = t9.*t12.*3.61307032511966e-6;
et46 = t10.*t12.*6.668858699921061e-6;
et47 = t12.*t14.*3.624676635982417e-6;
et48 = t10.*t157.*8.01825329916e-7+t14.*t157.*4.35810334311e-7;
et49 = t8.*t10.*t13.*(-3.624676635982417e-6);
et50 = t8.*t13.*t14.*6.668858699921061e-6;
et51 = t317+t321+t433+t473+t556+t574+t575+t597.*1.688944904408e-4-t598.*1.869599668e-7+t622+t623;
et52 = t680.*1.869599668e-7+t681.*1.688944904408e-4;
et53 = t9.*t772.*7.0482312e-7+t13.*t771.*7.0482312e-7+t246.*t777+t247.*t778+t294.*t775+t755.*(t119-t123);
et54 = t16.*t33.*t87.*4.563917575948183e-22;
et55 = t20.*t33.*t87.*(-7.086968837016952e-25);
et56 = t317+t321+t433+t473+t556+t574+t575+t604.*1.869599668e-7+t605.*1.688944904408e-4+t622+t623;
et57 = t9.*t752.*7.0482312e-7+t13.*t751.*7.0482312e-7+t246.*t758+t247.*t759+t294.*t757+t716.*(t119-t123);
et58 = t16.*t33.*t87.*1.279265104253459e-21;
et59 = t20.*t33.*t87.*(-1.6195873051144e-24);
et60 = t16.*(-2.706536467726674e-6);
et61 = t20.*6.078899754658124e-9-t13.*t16.*8.595599785252598e-9;
et62 = t13.*t176.*1.02e-6+t178.*t184+t176.*t187+t190.*t257-t9.*t499.*7.0482312e-7;
et63 = t13.*t500.*(-7.0482312e-7)+t246.*t538+t247.*t537-t294.*t579-t191.*(t53-t181)+t526.*(t119-t123);
et64 = 2.093791190610393e-6;
et65 = t9.*t17.*4.5672538176e-11;
et66 = t13.*t21.*1.020045672538176e-6+t17.*t184+t21.*t187+t80.*t246+t81.*t247+t183.*t294-t179.*(t119-t123)+t17.*t18.*t191+t17.*t22.*t190;
et67 = 4.097159105249182e-6;
et68 = t9.*4.0082304082032e-9;
et69 = t13.*1.87902861198544e-8-t18.*t190+t22.*t191+t180.*t294;
et70 = t13.*4.203395243364607e-6+t10.*t13.*8.01825329916e-7;
et71 = t13.*t14.*4.35810334311e-7;
et72 = t318+t440+t441+t474+t512+t513+t518+t522+t618+t621+t700.*1.35652563578e-4-t701.*6.1855407534e-5;
et73 = t734.*6.1855407534e-5+t735.*1.35652563578e-4+t338.*t775;
et74 = t318+t440+t441+t474+t512+t513+t518+t522+t618+t621+t634.*1.35652563578e-4-t635.*6.1855407534e-5;
et75 = t653.*6.1855407534e-5+t654.*1.35652563578e-4+t338.*t757;
et76 = t16.*(-2.289498402241797e-6);
et77 = t17.*2.048345525044518e-9;
et78 = t21.*9.602491515741889e-9;
et79 = t16.*t17.*(-3.086744386437578e-6);
et80 = t16.*t21.*(-6.769412826196288e-6);
et81 = t17.*t20.*1.615137793366553e-8;
et82 = t20.*t21.*(-3.445314443599436e-9)-t188.*t257-t338.*t579+t189.*(t53-t181);
et83 = t17.*4.0082304082032e-9;
et84 = t21.*1.87902861198544e-8+t183.*t338-t17.*t18.*t189-t17.*t22.*t188;
et85 = t439+t514+t571+t572+t739.*1.33637554986e-4+t740.*7.26350557185e-5;
et86 = t768.*7.26350557185e-5-t769.*1.33637554986e-4;
et87 = t439+t514+t571+t572+t655.*1.33637554986e-4+t656.*7.26350557185e-5;
et88 = t722.*(-1.33637554986e-4)+t723.*7.26350557185e-5;
et89 = t21.*2.148081562157245e-6;
et90 = t17.*t20.*3.61307032511966e-6;
et91 = t18.*t20.*6.668858699921061e-6;
et92 = t20.*t22.*3.624676635982417e-6;
et93 = t18.*t176.*8.01825329916e-7+t22.*t176.*4.35810334311e-7;
et94 = t16.*t18.*t21.*(-3.624676635982417e-6);
et95 = t16.*t21.*t22.*6.668858699921061e-6;
et96 = t21.*4.203395243364607e-6+t18.*t21.*8.01825329916e-7;
et97 = t21.*t22.*4.35810334311e-7;
mt1 = [t306+t424+t578+t590+t617+t642+t643+t674+t712+t718+t720+t596.*t627+t697.*t714+t699.*t715+t728.*t746+t747.*t749+t748.*t750+t755.*t756+t771.*t773+t772.*t774+t775.*t776+t777.*t779+t778.*t780+(t31-t38+2.243335e-2).*(et1+et2)+et3.*et4+2.377791947318098e-4];
mt2 = [et16+et17,et26+et27+et28,et51+et52+et53+et54+et55,et72+et73,et85+et86,et5+et6,et18+et19,t483+t497+t498+t525+t536+t584+t613+t628+t664+t665-t380.*t667+t381.*t669+t384.*t678+t583.*t716-t557.*t752+t585.*t758+t586.*t759-t624.*t757+t751.*(t218-t222-t235+t236),et56+et57+et58+et59,et74+et75,et87+et88,et7+et8,t278+t403+t481+t509+t581+t582+t626+t660+t670+t710+t711-t280.*t671+t281.*t672+t285.*t713-t499.*t754-t500.*t753+t526.*t729+t537.*t762+t538.*t761-t579.*t760,et29+et30+et31+et32,et60+et61+et62+et63+et64,et76+et77+et78+et79+et80+et81+et82,et89+et90+et91+et92+et93+et94+et95,et9+et10+et11+et12+et13,et20+et21+et22+et23,et33+et34+et35+et36,et65+et66+et67,et83+et84,et96+et97,et14+et15,et24+et25];
mt3 = [et37+et38+et39+et40+et41+et42+et43,et68+et69,t18.*t188-t22.*t189+t180.*t338+2.663570267859459e-6,0.0];
mt4 = [t434+t508+t565+t568+t10.*t763.*7.26350557185e-5-t14.*t763.*1.33637554986e-4+t114.*t732+t118.*t732];
mt5 = [t434+t508+t565+t568+t10.*t717.*7.26350557185e-5-t14.*t717.*1.33637554986e-4+t114.*t649+t118.*t649,et44+et45+et46+et47+et48+et49+et50,et70+et71,0.0];
mt6 = [4.203395243364607e-6];
H = reshape([mt1,mt2,mt3,mt4,mt5,mt6],6,6);
H = real(H);
end

== matlab function BDA_DynamicModel/Energy Analysis/MATLAB Function ==
  data: dq input; T output; H input
function T = Kinetic_Energy(dq, H)
T = real((1/2)*transpose(dq)*H*dq);

== matlab function BDA_DynamicModel/Energy Analysis/potential_energy ==
  data: q1 input; U output; q2 input; q3 input; q4 input; q5 input; q6 input
function U = potential_energy(q1,q2,q3,q4,q5,q6)
%#codegen

%    This function was generated by the Symbolic Math Toolbox version 9.0.
%    12-Oct-2021 13:17:17

t2 = conj(q1);
t3 = conj(q2);
t4 = conj(q3);
t5 = conj(q4);
t6 = conj(q5);
t7 = conj(q6);
t24 = 9.007199254740992e+15;
t8 = cos(t2);
t9 = cos(t3);
t10 = cos(t5);
t11 = cos(t6);
t12 = cos(t7);
t13 = sin(t2);
t14 = sin(t3);
t15 = sin(t5);
t16 = sin(t6);
t17 = sin(t7);
t18 = t2+t3;
t26 = (t4.*t24)./9.007199254740992e+15;
t29 = t4.*t24.*1.110223024625157e-16i;
t19 = cos(t18);
t20 = sin(t18);
t27 = cos(t26);
t28 = sin(t26);
t30 = -t29;
t31 = exp(t29);
t21 = t20.*4.602992943936994e+15;
t22 = t19.*7.742227997977903e+15;
t32 = -t27;
t33 = exp(t30);
t34 = t28.*1i;
t38 = t27.*7.38843356682345e-1;
t39 = t27.*2.61156643317655e-1;
t23 = -t21;
t35 = t33-1.0;
t37 = t27+t34;
t40 = t32+t34+1.0;
t42 = t10.*t24.*t28.*(t21-t22).*(-1.232595164407831e-32);
t43 = t15.*t24.*t28.*(t21-t22).*(-1.232595164407831e-32);
t44 = (t10.*t24.*t28.*(t21-t22))./8.112963841460668e+31;
t45 = t38+2.61156643317655e-1;
t46 = t39+7.38843356682345e-1;
t25 = t22+t23;
t36 = t35.^2;
t41 = t40.^2;
t47 = t19.*t45;
t48 = t20.*t46;
t49 = t20.*t37.*t41.*2.196325630278387e-1;
t50 = t19.*t37.*t41.*2.196325630278387e-1;
t51 = -t49;
t52 = -t50;
t53 = t47+t51;
t54 = t48+t52;
t55 = t10.*t54;
t56 = t11.*t53;
t57 = t15.*t54;
t58 = t43+t55;
t59 = t44+t57;
t60 = t16.*t59;
t61 = -t60;
t62 = t56+t61;
et1 = t8.*9.734313376175611e-2-t13.*2.717189118622151e-2;
et2 = t19.*3.161090981652867e-3+t20.*4.486342129859745e-3;
et3 = t47.*1.123016940370151e-2+t48.*9.0769442339979e-4;
et4 = t55.*1.663769266031448e-3+t56.*1.03455776890854e-3;
et5 = t57.*(-1.834077274308e-6)-t60.*1.03455776890854e-3;
et6 = t8.*t9.*1.805586507105727e-2;
et7 = t8.*t14.*2.789883597074818e-2;
et8 = t9.*t13.*2.789883597074818e-2;
et9 = t13.*t14.*(-1.805586507105727e-2);
et10 = t16.*t53.*1.33075164870018e-3+t11.*t59.*1.33075164870018e-3;
et11 = t12.*t58.*7.12549896598485e-4+t12.*t62.*1.31098441441266e-3;
et12 = t17.*t58.*(-1.31098441441266e-3)+t17.*t62.*7.12549896598485e-4;
et13 = t8.*t9.*t27.*7.73459091191916e-3;
et14 = t8.*t14.*t27.*(-4.598452461113469e-3);
et15 = t9.*t13.*t27.*(-4.598452461113469e-3);
et16 = t13.*t14.*t27.*(-7.73459091191916e-3);
et17 = t19.*t31.*t36.*(-1.993592526573721e-4);
et18 = t20.*t31.*t36.*(-1.027576994682181e-3);
et19 = t20.*t37.*t41.*(-1.438933894689597e-3);
et20 = t10.*t24.*t28.*(t21-t22).*(-2.260674779462336e-38);
et21 = t15.*t24.*t28.*(t21-t22).*(-2.050753952000729e-35);
U = real(et1+et2+et3+et4+et5+et6+et7+et8+et9+et10+et11+et12+et13+et14+et15+et16+et17+et18+et19+et20+et21);
